simulink model "TRABALHO"  (R2024a)
settings: Solver=VariableStepAuto  StartTime=0.0  StopTime=10.0  RelTol=1e-3
undefined symbols (not defined in the file or in its folder): A, Ak, B, b, Bk, C, Ck, Continuous, D, D1, D2, D3, H11, id, iq, J, K, Kdid, Kdidi, Kdiq, Kdiqi, Kdwi, Kqid, Kqidi, Kqiq, Kqiqi, Kqw, Kqwi, Kt, L, lamb, N, R, Time, Vd, Vq, w
libraries: ctrlSharedLib x1
settings Model: Creator=migue  LastModifiedBy=migue
settings DebuggingCC: UnconnectedInputMsg=warning  UnconnectedOutputMsg=warning  UnconnectedLineMsg=warning
settings ModelReferenceCC: EnableRefExpFcnMdlSchedulingChecks=on
settings RTWCC: GPUComputeCapability=3.5  DLArmComputeVersion=19.05

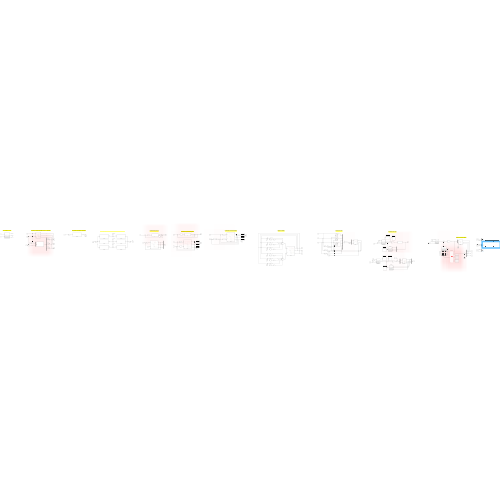
[thumbnail: Simulink's stored preview of the top-level diagram]
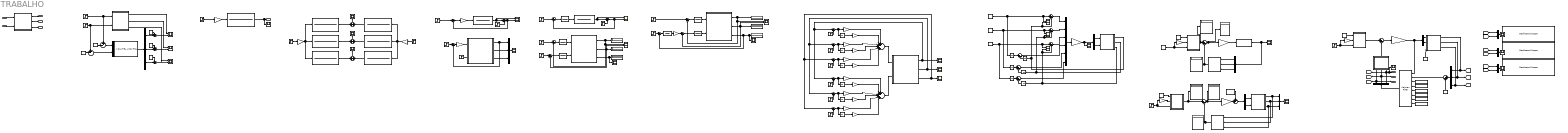
== system TRABALHO ==
  note: Checagem do LQR
  note: Espaço de estados
  note: Controlador Virtual de Velocidade
  note: Controlador Proporcional-Integrativo
  note: Controlador Proporcional
  note: Análise de proporcional controlando somente a velocidade no sistema
  note: Proporcional controlando a velocidade
  note: Comparação: Motor PMSM Não Lienar vs. Linearizada
  note: Motor PMSM Não Linear
  note: D1
  note: Controlador com LQR
  note: Malha com Filtro de Kalman
  In1 : Inport
  In2 : Inport  Port=2
  Add{1,3,6..11,13} (9 alike) : Sum  Inputs=|+-
  Add2 : Sum  Inputs=++|
  Add4 : Sum  Inputs=|++
  Aumentada : Subsystem
  Aumentada1 : Subsystem
  Aumentada2 : Subsystem
  Aumentada3 : Subsystem
  Aumentada6 : Subsystem
  Aumentada7 : Subsystem
  Constant : Constant  Value=Vd
  Constant1 : Constant  Value=Vq
  Constant10 : Constant
  Constant11 : Constant  Value=[0 0 150]
  Constant12 : Constant  Value=0
  Constant13 : Constant  Value=[0 0 0]
  Constant14 : Constant  Value=0
  Constant15 : Constant  Value=A
  Constant16 : Constant  Value=B
  Constant17 : Constant  Value=C
  Constant18 : Constant  Value=D
  Constant2 : Constant  Value=id
  Constant3 : Constant  Value=iq
  Constant4 : Constant  Value=w
  Constant5 : Constant  Value=id
  Constant6 : Constant  Value=iq
  Constant7 : Constant  Value=w
  Constant8 : Constant  Value=0
  Constant9 : Constant  Value=[Vd Vq]'
  D1 : TransferFcn  Numerator=D1.Numerator{:}  Denominator=D1.Denominator{:}
  D2 : TransferFcn  Numerator=D2.Numerator{:}  Denominator=D2.Denominator{:}
  D3 : TransferFcn  Numerator=D1.Numerator{:}  Denominator=D1.Denominator{:}
  D4 : TransferFcn  Numerator=D2.Numerator{:}.*[1 1000]  Denominator=D2.Denominator{:}
  D5 : TransferFcn  Numerator=D3.Numerator{:}  Denominator=D3.Denominator{:}
  Dashboard Scope : DashboardScope
  Dashboard Scope1 : DashboardScope
  Dashboard Scope2 : DashboardScope
  Demux : Demux  Outputs=3
  Demux1 : Demux  Outputs=3
  Demux2 : Demux  Outputs=3
  Demux3 : Demux  Outputs=2
  Demux4 : Demux  Outputs=2
  Demux5 : Demux  Outputs=2
  Display{,1..11} (12 alike) : Display
  Gain : Gain  Gain=7.35
  Gain1 : Gain  Gain=7.35
  Gain10 : Gain  Gain=Kqw
  Gain11 : Gain  Gain=Kqwi
  Gain12 : Gain  Gain=Kqw
  Gain13 : Gain  Gain=Kdwi
  Gain14 : Gain  Gain=Kqid
  Gain15 : Gain  Gain=Kqidi
  Gain16 : Gain  Gain=Kqiq
  Gain17 : Gain  Gain=Kqiqi
  Gain{18..20,25} (4 alike) : Gain  Gain=K  Multiplication=Matrix(K*u)
  Gain2 : Gain
  Gain21 : Gain  Gain=b/Kt
  Gain22 : Gain  Gain=b/Kt
  Gain26 : Gain  Gain=b/Kt
  Gain3 : Gain  Gain=0.265
  Gain4 : Gain  Gain=0.265
  Gain5 : Gain  Gain=1/Kt
  Gain6 : Gain  Gain=Kdid
  Gain7 : Gain  Gain=Kdidi
  Gain8 : Gain  Gain=Kdiq
  Gain9 : Gain  Gain=Kdiqi
  H1 : TransferFcn  Numerator=H11.Numerator{:}  Denominator=H11.Denominator{:}
  H11 : TransferFcn  Numerator=H11.Numerator{:}  Denominator=H11.Denominator{:}
  Id(S) [A] : Scope
  Id(s)/Vd(s) : TransferFcn  Numerator=[7692 9.468e6 2.295e1]  Denominator=[1 2462 6.748e6 3.672e9]
  Id(s)/Vq(s) : TransferFcn  Numerator=[1.154e7 1.282e6]  Denominator=[1 2462 6.748e6 3.672e9]
  Integrator{,1..11} (12 alike) : Integrator
  Iq(S) [A] : Scope
  Iq(s)/Vd(s) : TransferFcn  Numerator=[-1.154e7 -6.41e5]  Denominator=[1 2462 6.748e6 3.672e9]
  Iq(s)/Vq(s) : TransferFcn  Numerator=[7692 9.468e6 5.26e5]  Denominator=[1 2462 6.748e6 3.672e9]
  Kalman Filter1 : ctrlSharedLib/Kalman Filter  TimeDomain=Continuous-Time  UseCurrentEstimator=on  ModelSource=Input port  ModelSourceVariable=ss(0.95,1,1,0,1)  A=Ak  B=Bk  C=Ck  D=D  NumberOfStates=3  NumberOfInputs=2  NumberOfOutputs=3  InitialEstimateSource=Input port  X0=0  P0=10  UseK=off  UseGH=off  NumberOfProcessNoiseInputs=1  G=1  TimeInvariantG=on  H=0  TimeInvariantH=on  Q=0.05  TimeInvariantQ=on  R=1  TimeInvariantR=on  N=0  TimeInvariantN=on  AddInputPort=on  AddEnablePort=off  OutputEstimatedY=off  OutputP=off  Ts=-1
  Mux{,4,6..7} (4 alike) : Mux  Inputs=2
  Mux1 : Mux  Inputs=3
  Mux2 : Mux  Inputs=3
  Mux3 : Mux  Inputs=3
  Mux5 : Mux  Inputs=6
  PMSM : Subsystem  mask{R=0.16, L=1.3e-4, N=10, J=1.8e-4, b=1e-5, lamb=0.06, Kt=0.095}
      mask prompts: R "Resitência (R)"; L "Indutância(L)"; N "Nº de par de polos(N)"; J "coeficiente(J)"; b "coeficiente(b)"; lamb "(lamb)"; Kt "(Kt)"
  PMSM1 : Subsystem  mask{R=0.16, L=1.3e-4, N=10, J=1.8e-4, b=1e-5, lamb=0.06, Kt=0.095}
      mask prompts: R "Resitência (R)"; L "Indutância(L)"; N "Nº de par de polos(N)"; J "coeficiente(J)"; b "coeficiente(b)"; lamb "(lamb)"; Kt "(Kt)"
  PMSM2 : Subsystem  mask{R=0.16, L=1.3e-4, N=10, J=1.8e-4, b=1e-5, lamb=0.06, Kt=0.095}
      mask prompts: R "Resitência (R)"; L "Indutância(L)"; N "Nº de par de polos(N)"; J "coeficiente(J)"; b "coeficiente(b)"; lamb "(lamb)"; Kt "(Kt)"
  PMSM3 : Subsystem  mask{R=0.16, L=1.3e-4, N=10, J=1.8e-4, b=1e-5, lamb=0.06, Kt=0.095}
      mask prompts: R "Resitência (R)"; L "Indutância(L)"; N "Nº de par de polos(N)"; J "coeficiente(J)"; b "coeficiente(b)"; lamb "(lamb)"; Kt "(Kt)"
  PMSM5 : Subsystem  mask{R=0.16, L=1.3e-4, N=10, J=1.8e-4, b=1e-5, lamb=0.06, Kt=0.095}
      mask prompts: R "Resitência (R)"; L "Indutância(L)"; N "Nº de par de polos(N)"; J "coeficiente(J)"; b "coeficiente(b)"; lamb "(lamb)"; Kt "(Kt)"
  PMSM6 : Subsystem  mask{R=0.16, L=1.3e-4, N=10, J=1.8e-4, b=7.1808e-06, lamb=0.06, Kt=0.095}
      mask prompts: R "Resitência (R)"; L "Indutância(L)"; N "Nº de par de polos(N)"; J "coeficiente(J)"; b "coeficiente(b)"; lamb "(lamb)"; Kt "(Kt)"
  Random Number : RandomNumber  Variance=[0.1 0.1 5]  SampleTime=0.1
  Random Number1 : RandomNumber  Variance=[1 0.1 0.5]  SampleTime=0.1
  Scope{,1,4,7,11..13,15,18..23} (14 alike) : Scope
  Scope{2..3,5..6,8..10,14,16..17} (10 alike) : Scope  NumInputPorts=2
  State-Space : StateSpace  A=A  B=B  C=eye(3)  D=zeros(3,2)  InitialCondition=zeros(3,1)
  State-Space1 : StateSpace  A=A  B=B  C=eye(3)  D=zeros(3,2)  InitialCondition=zeros(3,1)
  Step : Step  Time=0.5  Before=Vd  After=Vd*1.1  SampleTime=0
  Step1 : Step  Time=0.5  Before=Vq  After=Vq*1.1  SampleTime=0
  Step{3,6,8,10,13..15} (7 alike) : Step  SampleTime=0
  Step11 : Step  Time=1.2  SampleTime=0
  Step12 : Step  After=0  SampleTime=0
  Step16 : Step  Before=150  After=151  SampleTime=0
  Step18 : Step  Before=150  After=151  SampleTime=0
  Step2 : Step  After=10  SampleTime=0
  Step4 : Step  Time=1.2  SampleTime=0
  Step5 : Step  Time=3  After=0  SampleTime=0
  Step7 : Step  Time=3  SampleTime=0
  Step9 : Step  After=100  SampleTime=0
  Subsystem : Subsystem  mask{R=0.16, L=1.3e-4, N=10, J=1.8e-4, b=1e-5, lamb=0.06, Kt=0.095}
      mask prompts: R "Resitência (R)"; L "Indutância(L)"; N "Nº de par de polos(N)"; J "coeficiente(J)"; b "coeficiente(b)"; lamb "(lamb)"; Kt "(Kt)"
  Subsystem1 : Subsystem  mask{R=0.16, L=1.3e-4, N=10, J=1.8e-4, b=1e-5, lamb=0.06, Kt=0.095}
      mask prompts: R "Resitência (R)"; L "Indutância(L)"; N "Nº de par de polos(N)"; J "coeficiente(J)"; b "coeficiente(b)"; lamb "(lamb)"; Kt "(Kt)"
  Subsystem2 : Subsystem
  Sum : Sum  Inputs=+-|
  Sum1 : Sum  Inputs=+-|
  Sum{8,10..12,14..17} (8 alike) : Sum  Inputs=|+-
  Sum13 : Sum  Inputs=|++
  Sum18 : Sum  Inputs=++++++|
  Sum{19..21,23..25} (6 alike) : Sum  Inputs=|-+
  Sum2 : Sum  Inputs=++|
  Sum22 : Sum  Inputs=++++++|
  Sum3 : Sum  Inputs=++|
  Sum4 : Sum  Inputs=++|
  Sum5 : Sum  Inputs=+|+
  Sum6 : Sum  Inputs=+|+
  Sum7 : Sum  Inputs=+|+
  Sum9 : Sum  Inputs=|++
  Transfer Fcn1 : TransferFcn  Numerator=D1.Numerator{:}  Denominator=D1.Denominator{:}
  Vd(S)1 : Step  After=0  SampleTime=0
  Vq(S) : Step  After=10  SampleTime=0
  W(S) : Scope
  W(s)/Vd(s) : TransferFcn  Numerator=[-6.09e9]  Denominator=[1 2462 6.748e6 3.672e9]
  W(s)/Vq(s) : TransferFcn  Numerator=[4.06e6 4.997e9]  Denominator=[1 2462 6.748e6 3.672e9]
  W(s)/Vq(s)1 : TransferFcn  Numerator=[4.06e6 4.997e9]  Denominator=[1 2462 6.748e6 3.672e9]
  idr : Step  SampleTime=0
  iqr : Step  SampleTime=0
  wr : Step  SampleTime=0
  Out1 : Outport
  Out2 : Outport  Port=2
  Out3 : Outport  Port=3
  Out4 : Outport  Port=4
  Out5 : Outport  Port=5
  Out6 : Outport  Port=6
  Out7 : Outport  Port=7
  wires:
  Demux/3 -> Sum4/2  "w~"
  Mux/1 -> State-Space/1
  Sum3/1 -> Scope8/2
  Sum4/1 -> Scope3/2
  State-Space/1 -> Demux/1
  Demux/2 -> Sum3/2  "iq~"
  Constant3/1 -> Sum3/1
  Constant4/1 -> Sum4/1
  Constant/1 -> Sum/2
  Subsystem/2(Iq) -> Scope8/1  "Iq"
  Demux/1 -> Sum2/2  "id~"
  Subsystem/1(Id) -> Scope9/1  "Id"
  Subsystem/3(w) -> Scope3/1  "w"
  Step/1 -> Sum/1, Subsystem/1(Vd)  "Vd"
  Sum/1 -> Mux/1  "Vd Linear"
  Sum1/1 -> Mux/2  "Vq Linear"
  Sum2/1 -> Scope9/2
  Constant2/1 -> Sum2/1
  Step1/1 -> Sum1/1, Subsystem/2(Vq)  "Vq"
  Constant1/1 -> Sum1/2
  W(s)/Vd(s)/1 -> Sum6/1  "[rad/s]"
  Id(s)/Vd(s)/1 -> Sum7/1  "[rad/s]"
  Iq(s)/Vd(s)/1 -> Sum5/1  "[rad/s]"
  Gain2/1 -> W(s)/Vd(s)/1, Iq(s)/Vd(s)/1, Id(s)/Vd(s)/1  "[V]"
  Iq(s)/Vq(s)/1 -> Sum5/2  "[rad/s]"
  Vd(S)1/1 -> Gain2/1
  Id(s)/Vq(s)/1 -> Sum7/2  "[rad/s]"
  Sum5/1 -> Iq(S) [A]/1
  W(s)/Vq(s)/1 -> Out4/1, Scope/1  "[rad/s]"
  W(s)/Vq(s)1/1 -> Sum6/2  "[rad/s]"
  Sum7/1 -> Id(S) [A]/1
  Gain1/1 -> Id(s)/Vq(s)/1, Iq(s)/Vq(s)/1, W(s)/Vq(s)1/1  "[V]"
  Vq(S)/1 -> Gain1/1
  Sum6/1 -> W(S)/1
  Gain/1 -> W(s)/Vq(s)/1  "[V]"
  Step2/1 -> Gain/1
  Mux1/1 -> Scope1/1
  Subsystem1/3(w) -> Mux1/3  "w"
  Step11/1 -> Subsystem1/2(Vq)
  Sum8/1 -> Gain3/1
  Sum10/1 -> Gain4/1
  Step4/1 -> Sum9/2
  Step10/1 -> Sum10/1
  H1/1 -> Scope2/1, Sum9/1
  Gain3/1 -> H1/1
  Subsystem1/2(Iq) -> Mux1/2  "Iq"
  Subsystem1/1(Id) -> Mux1/1, Sum10/2  "Id"
  Step3/1 -> Sum8/1
  Gain4/1 -> Subsystem1/1(Vd)
  Sum9/1 -> Sum8/2, Scope2/2
  Step6/1 -> Sum12/1
  PMSM/3(w) -> Scope4/1, Display2/1  "w"
  D2/1 -> PMSM/2(Vq)
  Step8/1 -> Sum14/1
  Sum12/1 -> Transfer Fcn1/1
  PMSM/1(Id) -> Display/1, Scope6/1, Sum14/2  "Id"
  Transfer Fcn1/1 -> H11/1
  D1/1 -> PMSM/1(Vd)
  Sum14/1 -> D1/1
  Step7/1 -> Sum13/2
  Sum13/1 -> Sum12/2, Scope5/2
  H11/1 -> Scope5/1, Sum13/1
  Sum11/1 -> D2/1
  Step5/1 -> Sum11/1
  PMSM/2(Iq) -> Display1/1, Scope6/2, Sum11/2  "Iq"
  D4/1 -> PMSM1/2(Vq)
  Gain5/1 -> Sum15/1
  PMSM1/2(Iq) -> Display4/1, Sum15/2, Scope10/2  "Iq"
  PMSM1/3(w) -> Scope7/1, Display5/1, Sum16/2  "w"
  Sum16/1 -> D5/1
  D5/1 -> Gain5/1
  Step9/1 -> Sum16/1
  Sum17/1 -> D3/1
  D3/1 -> PMSM1/1(Vd)
  Sum15/1 -> D4/1
  Step12/1 -> Sum17/1
  PMSM1/1(Id) -> Scope10/1, Sum17/2, Display3/1  "Id"
  Gain9/1 -> Sum18/4
  Sum18/1 -> PMSM2/1(Vd)
  Integrator/1 -> Gain7/1
  Sum24/1 -> Integrator4/1, Gain16/1
  iqr/1 -> Sum20/2
  Step15/1 -> Sum25/2
  PMSM2/2(Iq) -> Sum20/1, Sum24/1, Scope12/1  "Iq"
  Integrator4/1 -> Gain17/1
  Gain17/1 -> Sum22/4
  Gain15/1 -> Sum22/2
  Integrator5/1 -> Gain11/1
  Gain16/1 -> Sum22/3
  Integrator3/1 -> Gain15/1
  PMSM2/3(w) -> Scope13/1, Sum21/1, Sum25/1  "w"
  Sum23/1 -> Integrator3/1, Gain14/1
  Sum20/1 -> Integrator1/1, Gain8/1
  Gain13/1 -> Sum18/6
  idr/1 -> Sum19/2
  Sum25/1 -> Integrator5/1, Gain10/1
  Gain10/1 -> Sum22/5
  Gain6/1 -> Sum18/1
  Integrator1/1 -> Gain9/1
  Step13/1 -> Sum23/2
  Gain14/1 -> Sum22/1
  Gain11/1 -> Sum22/6
  Gain7/1 -> Sum18/2
  Gain12/1 -> Sum18/5
  Gain8/1 -> Sum18/3
  Sum19/1 -> Integrator/1, Gain6/1
  Step14/1 -> Sum24/2
  Sum21/1 -> Integrator2/1, Gain12/1
  Integrator2/1 -> Gain13/1
  PMSM2/1(Id) -> Scope11/1, Sum19/1, Sum23/1  "Id"
  wr/1 -> Sum21/2
  Sum22/1 -> PMSM2/2(Vq)
  Integrator9/1 -> Add11/2
  Mux5/1 -> Gain18/1
  Add10/1 -> Mux5/5
  Integrator7/1 -> Add10/1
  Add6/1 -> Mux5/1
  Constant6/1 -> Add7/1, Scope17/1, Integrator7/1  "iq"
  Demux3/2 -> PMSM3/2(Vq)
  Constant5/1 -> Integrator6/1, Add6/1, Scope14/1  "id"
  PMSM3/1(Id) -> Add6/2, Scope14/2, Integrator11/1  "Id"
  Add7/1 -> Mux5/2
  Demux3/1 -> PMSM3/1(Vd)
  PMSM3/3(w) -> Integrator9/1, Add8/2, Scope16/2  "w"
  Add8/1 -> Mux5/3
  Integrator8/1 -> Add11/1
  Constant7/1 -> Add8/1, Scope16/1, Integrator8/1  "w"
  Gain18/1 -> Scope15/1, Demux3/1
  Integrator6/1 -> Add9/1
  Add11/1 -> Mux5/6
  Integrator10/1 -> Add10/2
  Add9/1 -> Mux5/4
  PMSM3/2(Iq) -> Integrator10/1, Add7/2, Scope17/2  "Iq"
  Integrator11/1 -> Add9/2
  Aumentada3/1(Out1) -> Display8/1, Add1/1
  Aumentada2/1(Out1) -> Add1/2, Display7/1
  Constant10/1 -> Gain21/1, Aumentada3/3(w)  "w"
  Gain20/1 -> State-Space1/1
  Add1/1 -> Display6/1, Gain20/1
  Constant8/1 -> Aumentada3/1(Id)  "id"
  Demux1/2 -> Aumentada2/2(Iq)
  Demux1/3 -> Aumentada2/3(w)
  Demux1/1 -> Aumentada2/1(Id)
  State-Space1/1 -> Scope19/1, Demux1/1
  PMSM5/1(Id) -> Mux2/1, Aumentada/1(Id)  "Id"
  Aumentada1/1(Out1) -> Display10/1, Add3/1
  Aumentada/1(Out1) -> Display9/1, Add3/2
  PMSM5/2(Iq) -> Mux2/2, Aumentada/2(Iq)  "Iq"
  Demux4/1 -> PMSM5/1(Vd)
  Demux4/2 -> PMSM5/2(Vq)
  Mux2/1 -> Scope22/1
  PMSM5/3(w) -> Mux2/3, Aumentada/3(w)  "w"
  Add3/1 -> Display11/1, Gain19/1
  Gain21/1 -> Aumentada3/2(Iq)
  Add2/1 -> Demux4/1
  Gain19/1 -> Add2/2
  Constant9/1 -> Add2/1
  Constant12/1 -> Aumentada1/1(Id)  "id"
  Step16/1 -> Aumentada1/3(w), Gain22/1  "w"
  Gain22/1 -> Aumentada1/2(Iq)
  In1/1 -> Subsystem2/1(Vd)  "Vd"
  In2/1 -> Subsystem2/2(Vq)  "Vq"
  Subsystem2/1(Id) -> Out1/1
  Subsystem2/2(Iq) -> Out2/1
  Subsystem2/3(w) -> Out3/1
  PMSM6/1(Id) -> [idp], Mux3/1
  PMSM6/2(Iq) -> [iqp], Mux3/2  "Iq"
  Demux5/2 -> PMSM6/2(Vq)
  PMSM6/3(w) -> [wp], Mux3/3  "w"
  Demux5/1 -> PMSM6/1(Vd)
  Gain25/1 -> Demux5/1, Kalman Filter1/1
  Step18/1 -> Aumentada7/3(w), Gain26/1  "w"
  Gain26/1 -> Aumentada7/2(Iq)
  Constant14/1 -> Aumentada7/1(Id)  "id"
  Aumentada7/1(Out1) -> Add13/1
  Add13/1 -> Gain25/1
  Constant11/1 -> Kalman Filter1/3
  Constant13/1 -> Kalman Filter1/4
  Constant15/1 -> Kalman Filter1/5
  Constant16/1 -> Kalman Filter1/6
  Constant17/1 -> Kalman Filter1/7
  Constant18/1 -> Kalman Filter1/8
  Aumentada6/1(Out1) -> Add13/2
  Add4/1 -> Kalman Filter1/2
  Mux3/1 -> Add4/1
  Random Number/1 -> Add4/2
  Demux2/1 -> Aumentada6/1(Id), [idk], Out7/1
  Demux2/2 -> Aumentada6/2(Iq), Out6/1, [iqk]
  Demux2/3 -> Out5/1, Scope23/1, Aumentada6/3(w), [wk]
  Random Number1/1 -> PMSM6/3(In1)
  Kalman Filter1/1 -> Demux2/1
  Mux4/1 -> Scope18/1
  [wk] -> Mux4/1  "w filtrado"
  [wp] -> Mux4/2  "w saida"
  [idp] -> Mux6/2  "id saida"
  [idk] -> Mux6/1  "id filtrado"
  Mux6/1 -> Scope20/1
  Mux7/1 -> Scope21/1
  [iqk] -> Mux7/1  "iq filtrado"
  [iqp] -> Mux7/2  "iq saida"

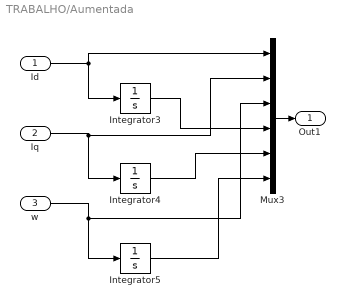
== system TRABALHO/Aumentada ==
  Id : Inport
  Iq : Inport  Port=2
  w : Inport  Port=3
  Integrator3 : Integrator
  Integrator4 : Integrator
  Integrator5 : Integrator
  Mux3 : Mux  Inputs=6
  Out1 : Outport
  wires:
  Iq/1 -> Mux3/2, Integrator4/1
  Id/1 -> Mux3/1, Integrator3/1
  w/1 -> Integrator5/1, Mux3/3
  Integrator3/1 -> Mux3/4
  Integrator5/1 -> Mux3/6
  Mux3/1 -> Out1/1
  Integrator4/1 -> Mux3/5

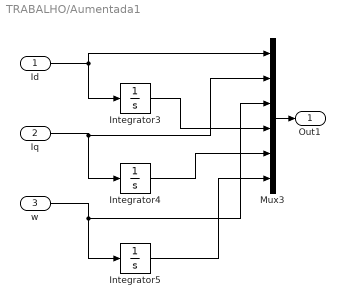
== system TRABALHO/Aumentada1 ==
  Id : Inport
  Iq : Inport  Port=2
  w : Inport  Port=3
  Integrator3 : Integrator
  Integrator4 : Integrator
  Integrator5 : Integrator
  Mux3 : Mux  Inputs=6
  Out1 : Outport
  wires:
  Iq/1 -> Mux3/2, Integrator4/1
  Id/1 -> Mux3/1, Integrator3/1
  w/1 -> Integrator5/1, Mux3/3
  Integrator3/1 -> Mux3/4
  Integrator5/1 -> Mux3/6
  Mux3/1 -> Out1/1
  Integrator4/1 -> Mux3/5

== system TRABALHO/Aumentada2 ==
  Id : Inport
  Iq : Inport  Port=2
  w : Inport  Port=3
  Integrator3 : Integrator
  Integrator4 : Integrator
  Integrator5 : Integrator
  Mux3 : Mux  Inputs=6
  Out1 : Outport
  wires:
  Iq/1 -> Mux3/2, Integrator4/1
  Id/1 -> Mux3/1, Integrator3/1
  w/1 -> Integrator5/1, Mux3/3
  Integrator3/1 -> Mux3/4
  Integrator5/1 -> Mux3/6
  Mux3/1 -> Out1/1
  Integrator4/1 -> Mux3/5

== system TRABALHO/Aumentada3 ==
  Id : Inport
  Iq : Inport  Port=2
  w : Inport  Port=3
  Integrator3 : Integrator
  Integrator4 : Integrator
  Integrator5 : Integrator
  Mux3 : Mux  Inputs=6
  Out1 : Outport
  wires:
  Iq/1 -> Mux3/2, Integrator4/1
  Id/1 -> Mux3/1, Integrator3/1
  w/1 -> Integrator5/1, Mux3/3
  Integrator3/1 -> Mux3/4
  Integrator5/1 -> Mux3/6
  Mux3/1 -> Out1/1
  Integrator4/1 -> Mux3/5

== system TRABALHO/Aumentada6 ==
  Id : Inport
  Iq : Inport  Port=2
  w : Inport  Port=3
  Integrator3 : Integrator
  Integrator4 : Integrator
  Integrator5 : Integrator
  Mux3 : Mux  Inputs=6
  Out1 : Outport
  wires:
  Iq/1 -> Mux3/2, Integrator4/1
  Id/1 -> Mux3/1, Integrator3/1
  w/1 -> Integrator5/1, Mux3/3
  Integrator3/1 -> Mux3/4
  Integrator5/1 -> Mux3/6
  Mux3/1 -> Out1/1
  Integrator4/1 -> Mux3/5

== system TRABALHO/Aumentada7 ==
  Id : Inport
  Iq : Inport  Port=2
  w : Inport  Port=3
  Integrator3 : Integrator
  Integrator4 : Integrator
  Integrator5 : Integrator
  Mux3 : Mux  Inputs=6
  Out1 : Outport
  wires:
  Iq/1 -> Mux3/2, Integrator4/1
  Id/1 -> Mux3/1, Integrator3/1
  w/1 -> Integrator5/1, Mux3/3
  Integrator3/1 -> Mux3/4
  Integrator5/1 -> Mux3/6
  Mux3/1 -> Out1/1
  Integrator4/1 -> Mux3/5

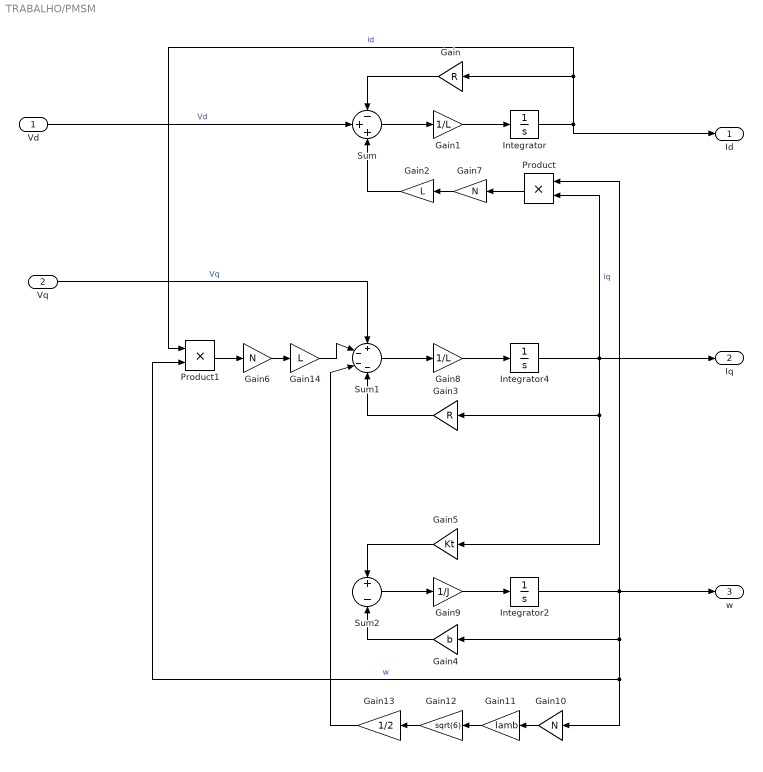
== system TRABALHO/PMSM ==
  Vd : Inport
  Vq : Inport  Port=2
  Gain : Gain  Gain=R
  Gain1 : Gain  Gain=1/L
  Gain10 : Gain  Gain=N
  Gain11 : Gain  Gain=lamb
  Gain12 : Gain  Gain=sqrt(6)
  Gain13 : Gain  Gain=1/2
  Gain14 : Gain  Gain=L
  Gain2 : Gain  Gain=L
  Gain3 : Gain  Gain=R
  Gain4 : Gain  Gain=b
  Gain5 : Gain  Gain=Kt
  Gain6 : Gain  Gain=N
  Gain7 : Gain  Gain=N
  Gain8 : Gain  Gain=1/L
  Gain9 : Gain  Gain=1/J
  Integrator : Integrator  InitialCondition=id
  Integrator2 : Integrator  InitialCondition=w
  Integrator4 : Integrator  InitialCondition=iq
  Product : Product
  Product1 : Product
  Sum : Sum  Inputs=-++
  Sum1 : Sum  Inputs=+---
  Sum2 : Sum  Inputs=+-
  Id : Outport
  Iq : Outport  Port=2
  w : Outport  Port=3
  wires:
  Integrator4/1 -> Iq/1, Product/2, Gain3/1, Gain5/1  "iq"
  Integrator/1 -> Gain/1, Product1/1, Id/1  "id"
  Gain8/1 -> Integrator4/1
  Sum1/1 -> Gain8/1
  Product1/1 -> Gain6/1
  Gain/1 -> Sum/1
  Sum2/1 -> Gain9/1
  Integrator2/1 -> w/1, Product/1, Gain10/1, Product1/2, Gain4/1  "w"
  Gain5/1 -> Sum2/1
  Vd/1 -> Sum/2  "Vd"
  Gain9/1 -> Integrator2/1
  Gain1/1 -> Integrator/1
  Sum/1 -> Gain1/1
  Gain4/1 -> Sum2/2
  Gain3/1 -> Sum1/4
  Gain11/1 -> Gain12/1
  Gain10/1 -> Gain11/1
  Product/1 -> Gain7/1
  Vq/1 -> Sum1/1  "Vq"
  Gain12/1 -> Gain13/1
  Gain13/1 -> Sum1/3
  Gain6/1 -> Gain14/1
  Gain7/1 -> Gain2/1
  Gain2/1 -> Sum/3
  Gain14/1 -> Sum1/2

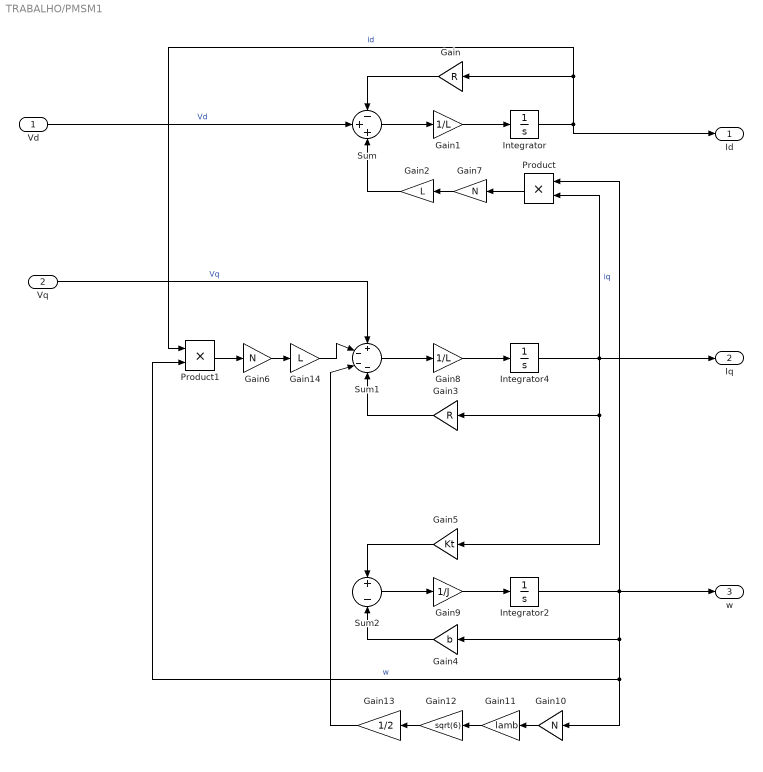
== system TRABALHO/PMSM1 ==
  Vd : Inport
  Vq : Inport  Port=2
  Gain : Gain  Gain=R
  Gain1 : Gain  Gain=1/L
  Gain10 : Gain  Gain=N
  Gain11 : Gain  Gain=lamb
  Gain12 : Gain  Gain=sqrt(6)
  Gain13 : Gain  Gain=1/2
  Gain14 : Gain  Gain=L
  Gain2 : Gain  Gain=L
  Gain3 : Gain  Gain=R
  Gain4 : Gain  Gain=b
  Gain5 : Gain  Gain=Kt
  Gain6 : Gain  Gain=N
  Gain7 : Gain  Gain=N
  Gain8 : Gain  Gain=1/L
  Gain9 : Gain  Gain=1/J
  Integrator : Integrator  InitialCondition=id
  Integrator2 : Integrator  InitialCondition=w
  Integrator4 : Integrator  InitialCondition=iq
  Product : Product
  Product1 : Product
  Sum : Sum  Inputs=-++
  Sum1 : Sum  Inputs=+---
  Sum2 : Sum  Inputs=+-
  Id : Outport
  Iq : Outport  Port=2
  w : Outport  Port=3
  wires:
  Integrator4/1 -> Iq/1, Product/2, Gain3/1, Gain5/1  "iq"
  Integrator/1 -> Gain/1, Product1/1, Id/1  "id"
  Gain8/1 -> Integrator4/1
  Sum1/1 -> Gain8/1
  Product1/1 -> Gain6/1
  Gain/1 -> Sum/1
  Sum2/1 -> Gain9/1
  Integrator2/1 -> w/1, Product/1, Gain10/1, Product1/2, Gain4/1  "w"
  Gain5/1 -> Sum2/1
  Vd/1 -> Sum/2  "Vd"
  Gain9/1 -> Integrator2/1
  Gain1/1 -> Integrator/1
  Sum/1 -> Gain1/1
  Gain4/1 -> Sum2/2
  Gain3/1 -> Sum1/4
  Gain11/1 -> Gain12/1
  Gain10/1 -> Gain11/1
  Product/1 -> Gain7/1
  Vq/1 -> Sum1/1  "Vq"
  Gain12/1 -> Gain13/1
  Gain13/1 -> Sum1/3
  Gain6/1 -> Gain14/1
  Gain7/1 -> Gain2/1
  Gain2/1 -> Sum/3
  Gain14/1 -> Sum1/2

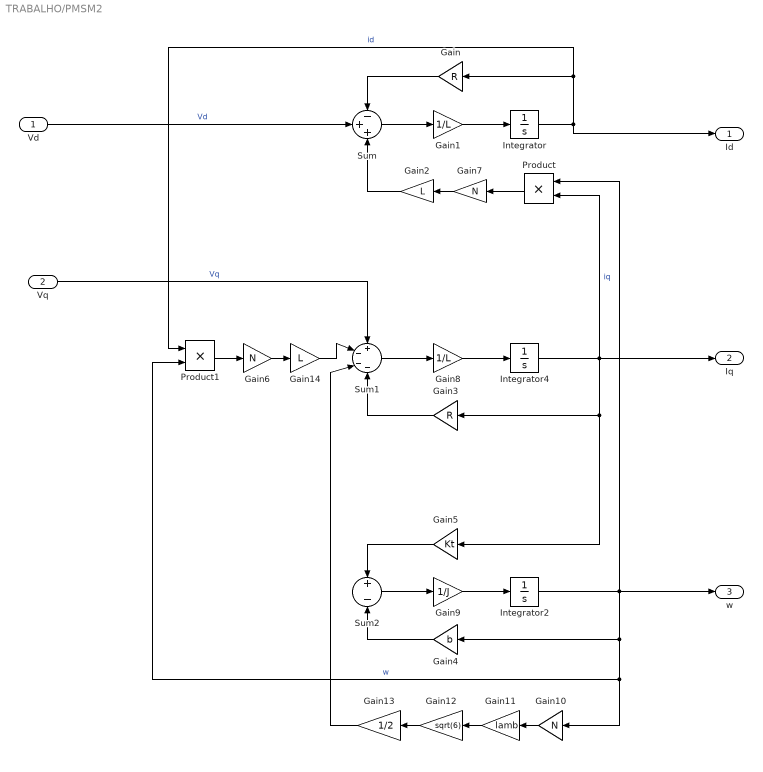
== system TRABALHO/PMSM2 ==
  Vd : Inport
  Vq : Inport  Port=2
  Gain : Gain  Gain=R
  Gain1 : Gain  Gain=1/L
  Gain10 : Gain  Gain=N
  Gain11 : Gain  Gain=lamb
  Gain12 : Gain  Gain=sqrt(6)
  Gain13 : Gain  Gain=1/2
  Gain14 : Gain  Gain=L
  Gain2 : Gain  Gain=L
  Gain3 : Gain  Gain=R
  Gain4 : Gain  Gain=b
  Gain5 : Gain  Gain=Kt
  Gain6 : Gain  Gain=N
  Gain7 : Gain  Gain=N
  Gain8 : Gain  Gain=1/L
  Gain9 : Gain  Gain=1/J
  Integrator : Integrator  InitialCondition=id
  Integrator2 : Integrator  InitialCondition=w
  Integrator4 : Integrator  InitialCondition=iq
  Product : Product
  Product1 : Product
  Sum : Sum  Inputs=-++
  Sum1 : Sum  Inputs=+---
  Sum2 : Sum  Inputs=+-
  Id : Outport
  Iq : Outport  Port=2
  w : Outport  Port=3
  wires:
  Integrator4/1 -> Iq/1, Product/2, Gain3/1, Gain5/1  "iq"
  Integrator/1 -> Gain/1, Product1/1, Id/1  "id"
  Gain8/1 -> Integrator4/1
  Sum1/1 -> Gain8/1
  Product1/1 -> Gain6/1
  Gain/1 -> Sum/1
  Sum2/1 -> Gain9/1
  Integrator2/1 -> w/1, Product/1, Gain10/1, Product1/2, Gain4/1  "w"
  Gain5/1 -> Sum2/1
  Vd/1 -> Sum/2  "Vd"
  Gain9/1 -> Integrator2/1
  Gain1/1 -> Integrator/1
  Sum/1 -> Gain1/1
  Gain4/1 -> Sum2/2
  Gain3/1 -> Sum1/4
  Gain11/1 -> Gain12/1
  Gain10/1 -> Gain11/1
  Product/1 -> Gain7/1
  Vq/1 -> Sum1/1  "Vq"
  Gain12/1 -> Gain13/1
  Gain13/1 -> Sum1/3
  Gain6/1 -> Gain14/1
  Gain7/1 -> Gain2/1
  Gain2/1 -> Sum/3
  Gain14/1 -> Sum1/2

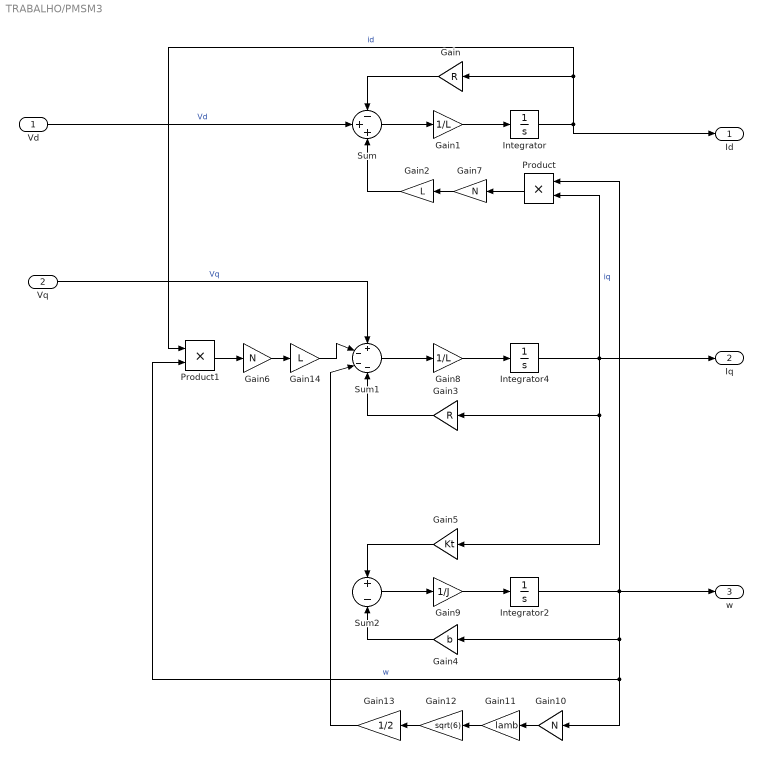
== system TRABALHO/PMSM3 ==
  Vd : Inport
  Vq : Inport  Port=2
  Gain : Gain  Gain=R
  Gain1 : Gain  Gain=1/L
  Gain10 : Gain  Gain=N
  Gain11 : Gain  Gain=lamb
  Gain12 : Gain  Gain=sqrt(6)
  Gain13 : Gain  Gain=1/2
  Gain14 : Gain  Gain=L
  Gain2 : Gain  Gain=L
  Gain3 : Gain  Gain=R
  Gain4 : Gain  Gain=b
  Gain5 : Gain  Gain=Kt
  Gain6 : Gain  Gain=N
  Gain7 : Gain  Gain=N
  Gain8 : Gain  Gain=1/L
  Gain9 : Gain  Gain=1/J
  Integrator : Integrator  InitialCondition=id
  Integrator2 : Integrator  InitialCondition=w
  Integrator4 : Integrator  InitialCondition=iq
  Product : Product
  Product1 : Product
  Sum : Sum  Inputs=-++
  Sum1 : Sum  Inputs=+---
  Sum2 : Sum  Inputs=+-
  Id : Outport
  Iq : Outport  Port=2
  w : Outport  Port=3
  wires:
  Integrator4/1 -> Iq/1, Product/2, Gain3/1, Gain5/1  "iq"
  Integrator/1 -> Gain/1, Product1/1, Id/1  "id"
  Gain8/1 -> Integrator4/1
  Sum1/1 -> Gain8/1
  Product1/1 -> Gain6/1
  Gain/1 -> Sum/1
  Sum2/1 -> Gain9/1
  Integrator2/1 -> w/1, Product/1, Gain10/1, Product1/2, Gain4/1  "w"
  Gain5/1 -> Sum2/1
  Vd/1 -> Sum/2  "Vd"
  Gain9/1 -> Integrator2/1
  Gain1/1 -> Integrator/1
  Sum/1 -> Gain1/1
  Gain4/1 -> Sum2/2
  Gain3/1 -> Sum1/4
  Gain11/1 -> Gain12/1
  Gain10/1 -> Gain11/1
  Product/1 -> Gain7/1
  Vq/1 -> Sum1/1  "Vq"
  Gain12/1 -> Gain13/1
  Gain13/1 -> Sum1/3
  Gain6/1 -> Gain14/1
  Gain7/1 -> Gain2/1
  Gain2/1 -> Sum/3
  Gain14/1 -> Sum1/2

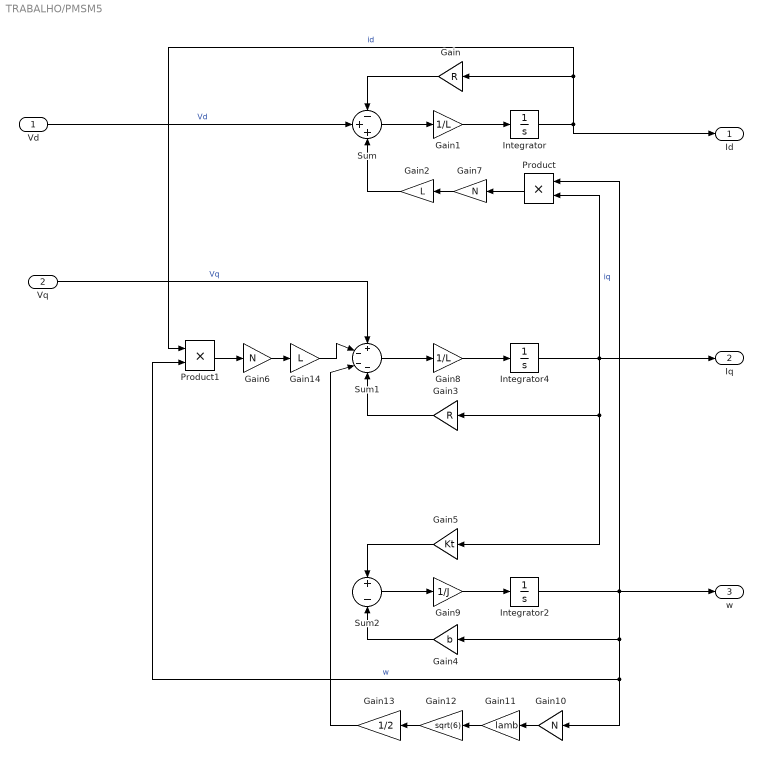
== system TRABALHO/PMSM5 ==
  Vd : Inport
  Vq : Inport  Port=2
  Gain : Gain  Gain=R
  Gain1 : Gain  Gain=1/L
  Gain10 : Gain  Gain=N
  Gain11 : Gain  Gain=lamb
  Gain12 : Gain  Gain=sqrt(6)
  Gain13 : Gain  Gain=1/2
  Gain14 : Gain  Gain=L
  Gain2 : Gain  Gain=L
  Gain3 : Gain  Gain=R
  Gain4 : Gain  Gain=b
  Gain5 : Gain  Gain=Kt
  Gain6 : Gain  Gain=N
  Gain7 : Gain  Gain=N
  Gain8 : Gain  Gain=1/L
  Gain9 : Gain  Gain=1/J
  Integrator : Integrator  InitialCondition=id
  Integrator2 : Integrator  InitialCondition=w
  Integrator4 : Integrator  InitialCondition=iq
  Product : Product
  Product1 : Product
  Sum : Sum  Inputs=-++
  Sum1 : Sum  Inputs=+---
  Sum2 : Sum  Inputs=+-
  Id : Outport
  Iq : Outport  Port=2
  w : Outport  Port=3
  wires:
  Integrator4/1 -> Iq/1, Product/2, Gain3/1, Gain5/1  "iq"
  Integrator/1 -> Gain/1, Product1/1, Id/1  "id"
  Gain8/1 -> Integrator4/1
  Sum1/1 -> Gain8/1
  Product1/1 -> Gain6/1
  Gain/1 -> Sum/1
  Sum2/1 -> Gain9/1
  Integrator2/1 -> w/1, Product/1, Gain10/1, Product1/2, Gain4/1  "w"
  Gain5/1 -> Sum2/1
  Vd/1 -> Sum/2  "Vd"
  Gain9/1 -> Integrator2/1
  Gain1/1 -> Integrator/1
  Sum/1 -> Gain1/1
  Gain4/1 -> Sum2/2
  Gain3/1 -> Sum1/4
  Gain11/1 -> Gain12/1
  Gain10/1 -> Gain11/1
  Product/1 -> Gain7/1
  Vq/1 -> Sum1/1  "Vq"
  Gain12/1 -> Gain13/1
  Gain13/1 -> Sum1/3
  Gain6/1 -> Gain14/1
  Gain7/1 -> Gain2/1
  Gain2/1 -> Sum/3
  Gain14/1 -> Sum1/2

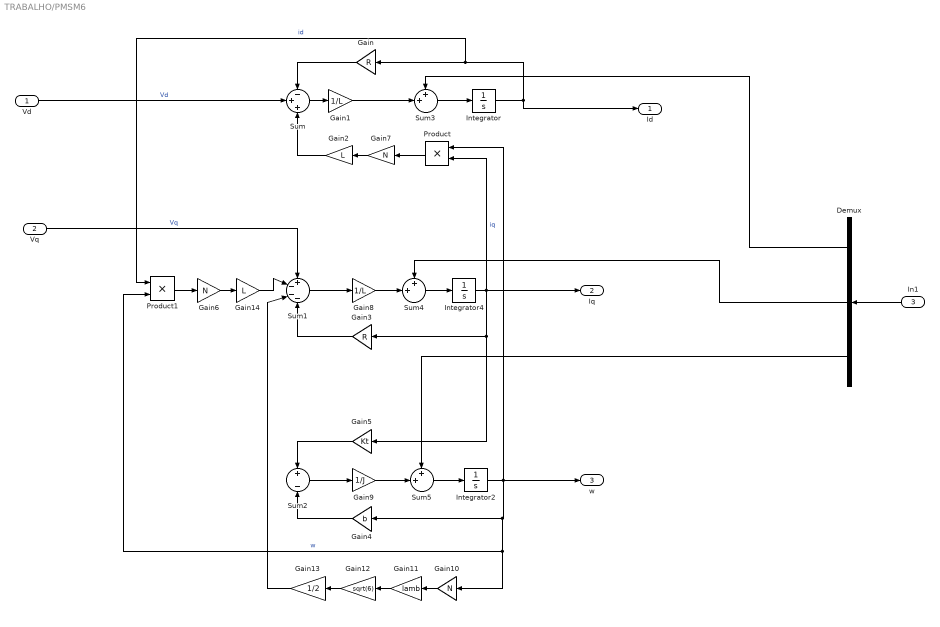
== system TRABALHO/PMSM6 ==
  Vd : Inport
  Vq : Inport  Port=2
  In1 : Inport  Port=3
  Demux : Demux  Outputs=3
  Gain : Gain  Gain=R
  Gain1 : Gain  Gain=1/L
  Gain10 : Gain  Gain=N
  Gain11 : Gain  Gain=lamb
  Gain12 : Gain  Gain=sqrt(6)
  Gain13 : Gain  Gain=1/2
  Gain14 : Gain  Gain=L
  Gain2 : Gain  Gain=L
  Gain3 : Gain  Gain=R
  Gain4 : Gain  Gain=b
  Gain5 : Gain  Gain=Kt
  Gain6 : Gain  Gain=N
  Gain7 : Gain  Gain=N
  Gain8 : Gain  Gain=1/L
  Gain9 : Gain  Gain=1/J
  Integrator : Integrator  InitialCondition=id
  Integrator2 : Integrator  InitialCondition=w
  Integrator4 : Integrator  InitialCondition=iq
  Product : Product
  Product1 : Product
  Sum : Sum  Inputs=-++
  Sum1 : Sum  Inputs=+---
  Sum2 : Sum  Inputs=+-
  Sum3 : Sum  Inputs=++|
  Sum4 : Sum  Inputs=++|
  Sum5 : Sum  Inputs=++|
  Id : Outport
  Iq : Outport  Port=2
  w : Outport  Port=3
  wires:
  Integrator4/1 -> Iq/1, Product/2, Gain3/1, Gain5/1  "iq"
  Integrator/1 -> Gain/1, Product1/1, Id/1  "id"
  Sum1/1 -> Gain8/1
  Product1/1 -> Gain6/1
  Gain/1 -> Sum/1
  Sum2/1 -> Gain9/1
  Integrator2/1 -> w/1, Product/1, Gain10/1, Product1/2, Gain4/1  "w"
  Gain5/1 -> Sum2/1
  Vd/1 -> Sum/2  "Vd"
  Sum/1 -> Gain1/1
  Gain4/1 -> Sum2/2
  Gain3/1 -> Sum1/4
  Gain11/1 -> Gain12/1
  Gain10/1 -> Gain11/1
  Product/1 -> Gain7/1
  Vq/1 -> Sum1/1  "Vq"
  Gain12/1 -> Gain13/1
  Gain13/1 -> Sum1/3
  Gain6/1 -> Gain14/1
  Gain7/1 -> Gain2/1
  Gain2/1 -> Sum/3
  Gain14/1 -> Sum1/2
  Gain1/1 -> Sum3/2
  Sum3/1 -> Integrator/1
  Sum4/1 -> Integrator4/1
  Gain8/1 -> Sum4/2
  Sum5/1 -> Integrator2/1
  Gain9/1 -> Sum5/2
  Demux/1 -> Sum3/1
  Demux/2 -> Sum4/1
  Demux/3 -> Sum5/1
  In1/1 -> Demux/1

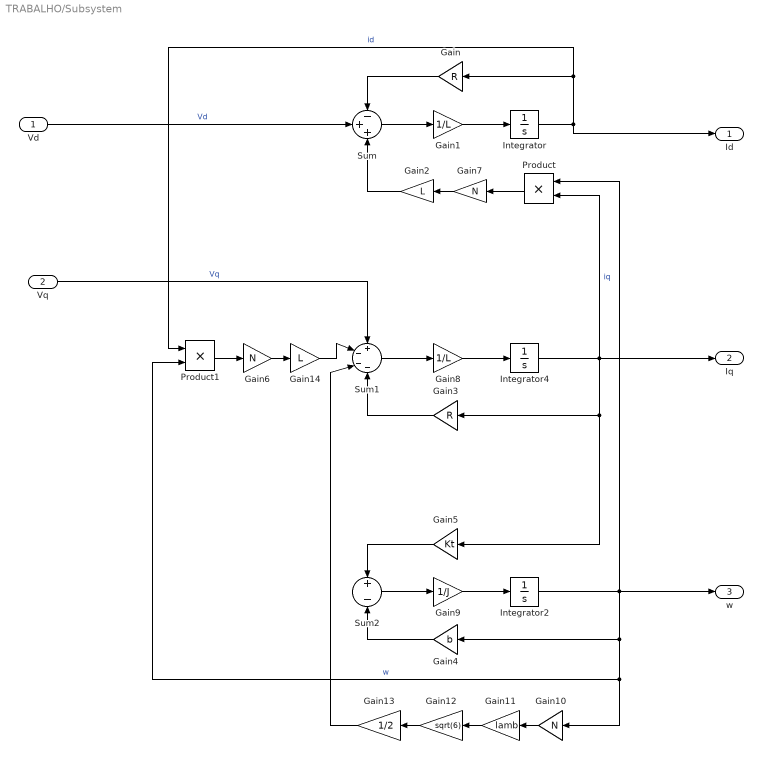
== system TRABALHO/Subsystem ==
  Vd : Inport
  Vq : Inport  Port=2
  Gain : Gain  Gain=R
  Gain1 : Gain  Gain=1/L
  Gain10 : Gain  Gain=N
  Gain11 : Gain  Gain=lamb
  Gain12 : Gain  Gain=sqrt(6)
  Gain13 : Gain  Gain=1/2
  Gain14 : Gain  Gain=L
  Gain2 : Gain  Gain=L
  Gain3 : Gain  Gain=R
  Gain4 : Gain  Gain=b
  Gain5 : Gain  Gain=Kt
  Gain6 : Gain  Gain=N
  Gain7 : Gain  Gain=N
  Gain8 : Gain  Gain=1/L
  Gain9 : Gain  Gain=1/J
  Integrator : Integrator  InitialCondition=id
  Integrator2 : Integrator  InitialCondition=w
  Integrator4 : Integrator  InitialCondition=iq
  Product : Product
  Product1 : Product
  Sum : Sum  Inputs=-++
  Sum1 : Sum  Inputs=+---
  Sum2 : Sum  Inputs=+-
  Id : Outport
  Iq : Outport  Port=2
  w : Outport  Port=3
  wires:
  Integrator4/1 -> Iq/1, Product/2, Gain3/1, Gain5/1  "iq"
  Integrator/1 -> Gain/1, Product1/1, Id/1  "id"
  Gain8/1 -> Integrator4/1
  Sum1/1 -> Gain8/1
  Product1/1 -> Gain6/1
  Gain/1 -> Sum/1
  Sum2/1 -> Gain9/1
  Integrator2/1 -> w/1, Product/1, Gain10/1, Product1/2, Gain4/1  "w"
  Gain5/1 -> Sum2/1
  Vd/1 -> Sum/2  "Vd"
  Gain9/1 -> Integrator2/1
  Gain1/1 -> Integrator/1
  Sum/1 -> Gain1/1
  Gain4/1 -> Sum2/2
  Gain3/1 -> Sum1/4
  Gain11/1 -> Gain12/1
  Gain10/1 -> Gain11/1
  Product/1 -> Gain7/1
  Vq/1 -> Sum1/1  "Vq"
  Gain12/1 -> Gain13/1
  Gain13/1 -> Sum1/3
  Gain6/1 -> Gain14/1
  Gain7/1 -> Gain2/1
  Gain2/1 -> Sum/3
  Gain14/1 -> Sum1/2

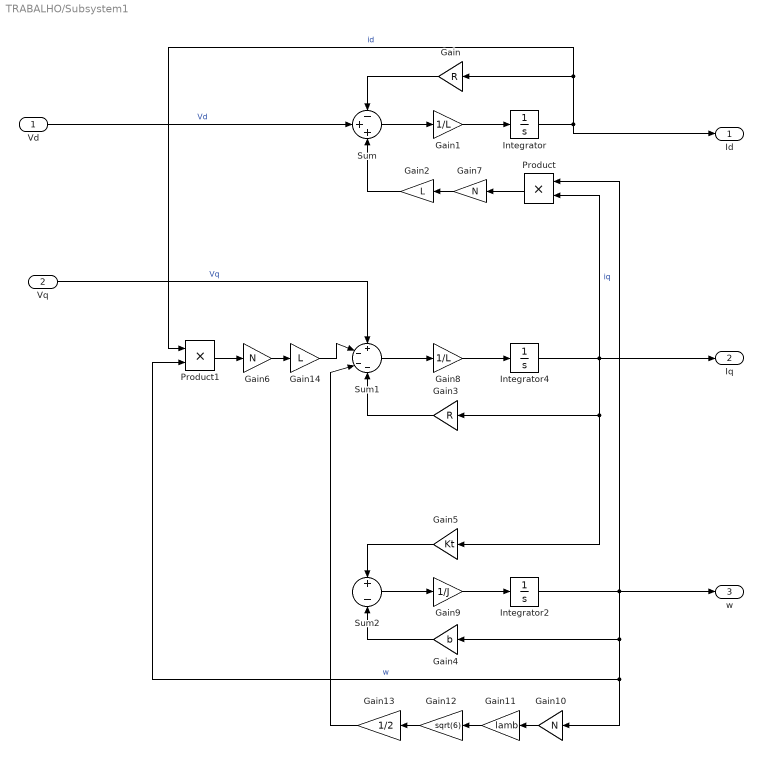
== system TRABALHO/Subsystem1 ==
  Vd : Inport
  Vq : Inport  Port=2
  Gain : Gain  Gain=R
  Gain1 : Gain  Gain=1/L
  Gain10 : Gain  Gain=N
  Gain11 : Gain  Gain=lamb
  Gain12 : Gain  Gain=sqrt(6)
  Gain13 : Gain  Gain=1/2
  Gain14 : Gain  Gain=L
  Gain2 : Gain  Gain=L
  Gain3 : Gain  Gain=R
  Gain4 : Gain  Gain=b
  Gain5 : Gain  Gain=Kt
  Gain6 : Gain  Gain=N
  Gain7 : Gain  Gain=N
  Gain8 : Gain  Gain=1/L
  Gain9 : Gain  Gain=1/J
  Integrator : Integrator  InitialCondition=id
  Integrator2 : Integrator  InitialCondition=w
  Integrator4 : Integrator  InitialCondition=iq
  Product : Product
  Product1 : Product
  Sum : Sum  Inputs=-++
  Sum1 : Sum  Inputs=+---
  Sum2 : Sum  Inputs=+-
  Id : Outport
  Iq : Outport  Port=2
  w : Outport  Port=3
  wires:
  Integrator4/1 -> Iq/1, Product/2, Gain3/1, Gain5/1  "iq"
  Integrator/1 -> Gain/1, Product1/1, Id/1  "id"
  Gain8/1 -> Integrator4/1
  Sum1/1 -> Gain8/1
  Product1/1 -> Gain6/1
  Gain/1 -> Sum/1
  Sum2/1 -> Gain9/1
  Integrator2/1 -> w/1, Product/1, Gain10/1, Product1/2, Gain4/1  "w"
  Gain5/1 -> Sum2/1
  Vd/1 -> Sum/2  "Vd"
  Gain9/1 -> Integrator2/1
  Gain1/1 -> Integrator/1
  Sum/1 -> Gain1/1
  Gain4/1 -> Sum2/2
  Gain3/1 -> Sum1/4
  Gain11/1 -> Gain12/1
  Gain10/1 -> Gain11/1
  Product/1 -> Gain7/1
  Vq/1 -> Sum1/1  "Vq"
  Gain12/1 -> Gain13/1
  Gain13/1 -> Sum1/3
  Gain6/1 -> Gain14/1
  Gain7/1 -> Gain2/1
  Gain2/1 -> Sum/3
  Gain14/1 -> Sum1/2

== system TRABALHO/Subsystem2 ==
  Vd : Inport
  Vq : Inport  Port=2
  " PMSM " : Subsystem  Commented=on
  Id : Outport
  Iq : Outport  Port=2
  w : Outport  Port=3
  wires:
  " PMSM "/1(Id) -> Id/1
  " PMSM "/2(Iq) -> Iq/1
  " PMSM "/3(w) -> w/1
  Vq/1 -> " PMSM "/2(Vq)
  Vd/1 -> " PMSM "/1(Vd)

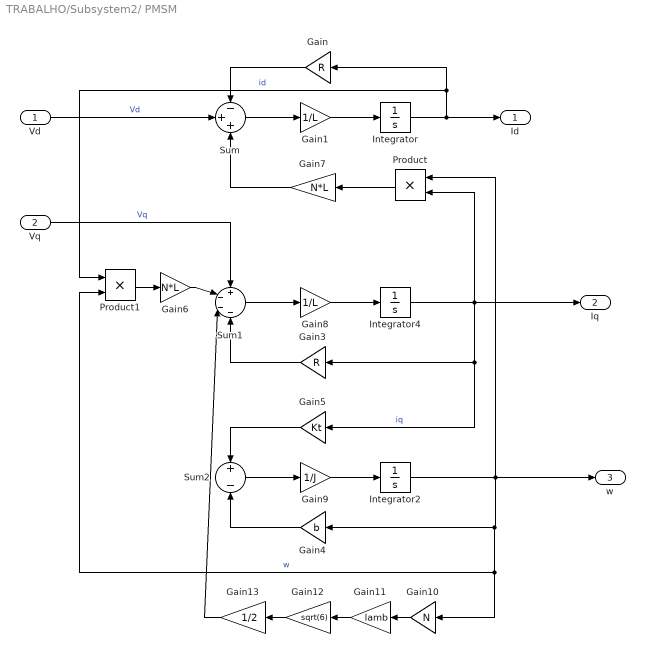
== system TRABALHO/Subsystem2/ PMSM  ==
  Vd : Inport
  Vq : Inport  Port=2
  Gain : Gain  Gain=R
  Gain1 : Gain  Gain=1/L
  Gain10 : Gain  Gain=N
  Gain11 : Gain  Gain=lamb
  Gain12 : Gain  Gain=sqrt(6)
  Gain13 : Gain  Gain=1/2
  Gain3 : Gain  Gain=R
  Gain4 : Gain  Gain=b
  Gain5 : Gain  Gain=Kt
  Gain6 : Gain  Gain=N*L
  Gain7 : Gain  Gain=N*L
  Gain8 : Gain  Gain=1/L
  Gain9 : Gain  Gain=1/J
  Integrator : Integrator
  Integrator2 : Integrator
  Integrator4 : Integrator
  Product : Product
  Product1 : Product
  Sum : Sum  Inputs=-++
  Sum1 : Sum  Inputs=+---
  Sum2 : Sum  Inputs=+-
  Id : Outport
  Iq : Outport  Port=2
  w : Outport  Port=3
  wires:
  Integrator4/1 -> Iq/1, Product/2, Gain3/1, Gain5/1  "iq"
  Integrator/1 -> Id/1, Gain/1, Product1/1  "id"
  Gain8/1 -> Integrator4/1
  Sum1/1 -> Gain8/1
  Product1/1 -> Gain6/1
  Gain/1 -> Sum/1
  Sum2/1 -> Gain9/1
  Integrator2/1 -> w/1, Product/1, Gain10/1, Product1/2, Gain4/1  "w"
  Gain5/1 -> Sum2/1
  Vd/1 -> Sum/2  "Vd"
  Gain9/1 -> Integrator2/1
  Gain1/1 -> Integrator/1
  Sum/1 -> Gain1/1
  Gain4/1 -> Sum2/2
  Gain3/1 -> Sum1/4
  Gain11/1 -> Gain12/1
  Gain10/1 -> Gain11/1
  Product/1 -> Gain7/1
  Vq/1 -> Sum1/1  "Vq"
  Gain12/1 -> Gain13/1
  Gain13/1 -> Sum1/3
  Gain6/1 -> Sum1/2
  Gain7/1 -> Sum/3
